simulink model "Octacopter_Model_24b"  (R2025b)
settings: Solver=VariableStepAuto  StartTime=0.0  StopTime=10  RelTol=1e-3
values from neighbouring files (symbols this model uses):
  Alt = 600    [Octa_Initialise.m]
  c = -500    [Octa_Initialise.m]
  Drag_on = 1    [Octa_Initialise.m]
  g = 9.81    [Octa_Initialise.m]
  I = [I_xx, I_xy, I_xz; I_xy, I_yy, I_yz; I_xz, I_yz, I_zz]    [Octa_Initialise.m]
  I_xx = 0.35    [Octa_Initialise.m]
  I_yy = 0.35    [Octa_Initialise.m]
  I_zz = 0.67    [Octa_Initialise.m]
  k = 6500    [Octa_Initialise.m]
  k_D = [0.05, 0.05, 0.15]    [Octa_Initialise.m]
  k_q = (Cp*Rho*(D)^5)/(8*(pi)^3)    (= 1.08765022525e-07)    [Octa_Initialise.m]
  l_arm1 = [l*cosd(0) l*sind(0) 0]    [Octa_Initialise.m]
  l_arm2 = [l*cosd(-45) l*sind(-45) 0]    [Octa_Initialise.m]
  l_arm3 = [l*cosd(-90) l*sind(-90) 0]    [Octa_Initialise.m]
  l_arm4 = [l*cosd(-135) l*sind(-135) 0]    [Octa_Initialise.m]
  l_arm5 = [l*cosd(-180) l*sind(-180) 0]    [Octa_Initialise.m]
  l_arm6 = [l*cosd(135) l*sind(135) 0]    [Octa_Initialise.m]
  l_arm7 = [l*cosd(90) l*sind(90) 0]    [Octa_Initialise.m]
  l_arm8 = [l*cosd(45) l*sind(45) 0]    [Octa_Initialise.m]
  m = 6.71    [Octa_Initialise.m]
  M1_set_phi = 0    [Octa_Initialise.m]
  M1_set_theta = 0    [Octa_Initialise.m]
  M2_set_phi = 0    [Octa_Initialise.m]
  M2_set_theta = 0    [Octa_Initialise.m]
  M3_set_phi = 0    [Octa_Initialise.m]
  M3_set_theta = 0    [Octa_Initialise.m]
  M4_set_phi = 0    [Octa_Initialise.m]
  M4_set_theta = 0    [Octa_Initialise.m]
  M5_set_phi = 0    [Octa_Initialise.m]
  M5_set_theta = 0    [Octa_Initialise.m]
  M6_set_phi = 0    [Octa_Initialise.m]
  M6_set_theta = 0    [Octa_Initialise.m]
  M7_set_phi = 0    [Octa_Initialise.m]
  M7_set_theta = 0    [Octa_Initialise.m]
  M8_set_phi = 0    [Octa_Initialise.m]
  M8_set_theta = 0    [Octa_Initialise.m]
  p_dot_dot_0 = 0    [Octa_Initialise.m]
  phi_dot_0 = phi_theta_psi_dot_0(1)    [Octa_Initialise.m]
  phi_lower = deg2rad(-180)    [Octa_Initialise.m]
  phi_upper = deg2rad(180)    [Octa_Initialise.m]
  psi_dot_0 = phi_theta_psi_dot_0(3)    [Octa_Initialise.m]
  q_dot_dot_0 = 0    [Octa_Initialise.m]
  r_dot_dot_0 = 0    [Octa_Initialise.m]
  rpm2rad_s = pi/30    (= 0.10471975512)    [Octa_Initialise.m]
  RPM_max = 17668    [Octa_Initialise.m]    (also in Thrust_Plots.m = 15000)
  RPM_min = 0    [Octa_Initialise.m]    (also in Thrust_Plots.m)
  Tau_ESC1 = 0.15    [Octa_Initialise.m]
  Tau_ESC2 = 0.15    [Octa_Initialise.m]
  Tau_ESC3 = 0.15    [Octa_Initialise.m]
  Tau_ESC4 = 0.15    [Octa_Initialise.m]
  Tau_ESC5 = 0.15    [Octa_Initialise.m]
  Tau_ESC6 = 0.15    [Octa_Initialise.m]
  Tau_ESC7 = 0.15    [Octa_Initialise.m]
  Tau_ESC8 = 0.15    [Octa_Initialise.m]
  theta_dot_0 = phi_theta_psi_dot_0(2)    [Octa_Initialise.m]
  theta_lower = deg2rad(-90)    [Octa_Initialise.m]
  theta_upper = deg2rad(90)    [Octa_Initialise.m]
  Thrust_max = 20    [Octa_Initialise.m]
  thrustData = load('Cine66 Thrust Params.mat')    [Thrust_Plots.m]
  u_0 = u_v_w_0(1)    [Octa_Initialise.m]
  u_dot_0 = 0    [Octa_Initialise.m]
  v_0 = u_v_w_0(2)    [Octa_Initialise.m]
  v_dot_0 = 0    [Octa_Initialise.m]
  w1_0 = 0    [Octa_Initialise.m]
  w2_0 = 0    [Octa_Initialise.m]
  w3_0 = 0    [Octa_Initialise.m]
  w4_0 = 0    [Octa_Initialise.m]
  w5_0 = 0    [Octa_Initialise.m]
  w6_0 = 0    [Octa_Initialise.m]
  w7_0 = 0    [Octa_Initialise.m]
  w8_0 = 0    [Octa_Initialise.m]
  w_0 = u_v_w_0(3)    [Octa_Initialise.m]
  w_d_1 = -1    [Octa_Initialise.m]
  w_d_2 = +1.    (= 1)    [Octa_Initialise.m]
  w_d_3 = -1    [Octa_Initialise.m]
  w_d_4 = +1    (= 1)    [Octa_Initialise.m]
  w_d_5 = -1    [Octa_Initialise.m]
  w_d_6 = +1    (= 1)    [Octa_Initialise.m]
  w_d_7 = -1    [Octa_Initialise.m]
  w_d_8 = +1    (= 1)    [Octa_Initialise.m]
  w_dot_0 = 0    [Octa_Initialise.m]
undefined symbols (not defined in the file or in its folder): DiscIntNeverNeededParam
libraries: matrix_library x10, simulink x3, px4uORBlib x1, aerolibutil x1, px4Peripheralslib x1
(part 1 of 2)
settings Model: PauseTimes=0.1  Creator=Admin  LastModifiedBy=Admin
settings DebuggingCC: AlgebraicLoopMsg=none

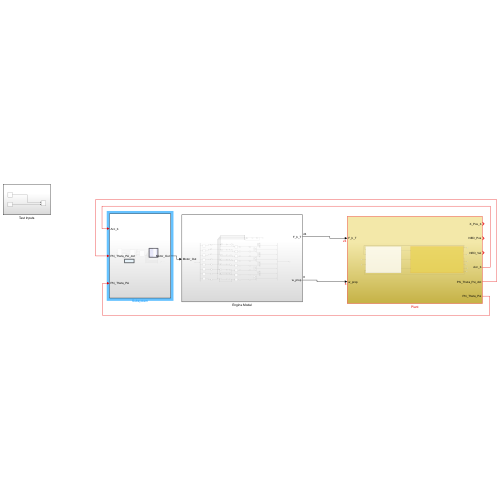
[thumbnail: Simulink's stored preview of the top-level diagram]
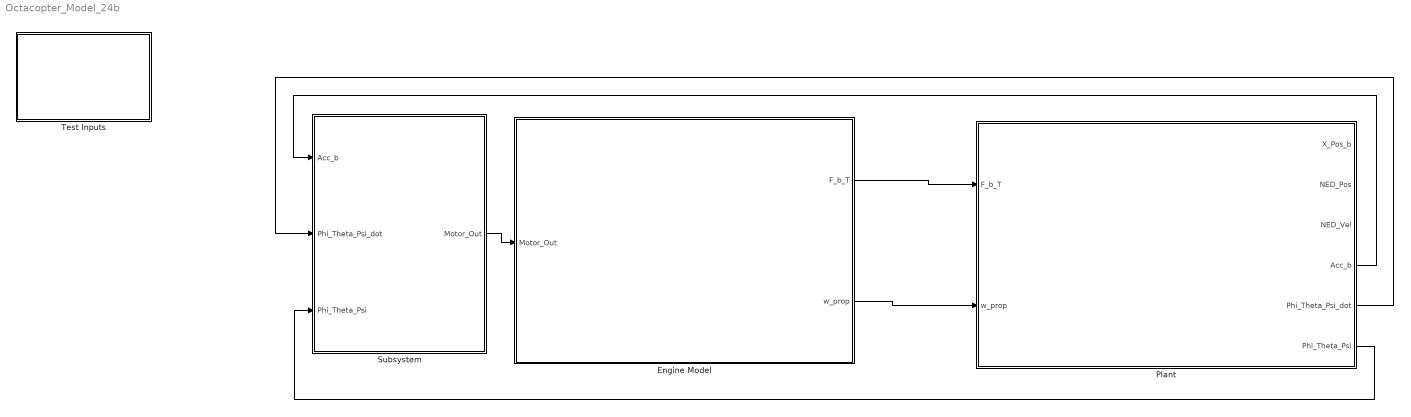
== system Octacopter_Model_24b ==
  Engine Model : Subsystem
  Plant : Subsystem
  Subsystem : Subsystem
  Test Inputs : Subsystem
  wires:
  Engine Model/1(F_b_T) -> Plant/1(F_b_T)
  Engine Model/2(w_prop) -> Plant/2(w_prop)
  Subsystem/1(Motor_Out) -> Engine Model/1(Motor_Out)
  Plant/4(Acc_b) -> Subsystem/1(Acc_b)
  Plant/5(Phi_Theta_Psi_dot) -> Subsystem/2(Phi_Theta_Psi_dot)
  Plant/6(Phi_Theta_Psi) -> Subsystem/3(Phi_Theta_Psi)

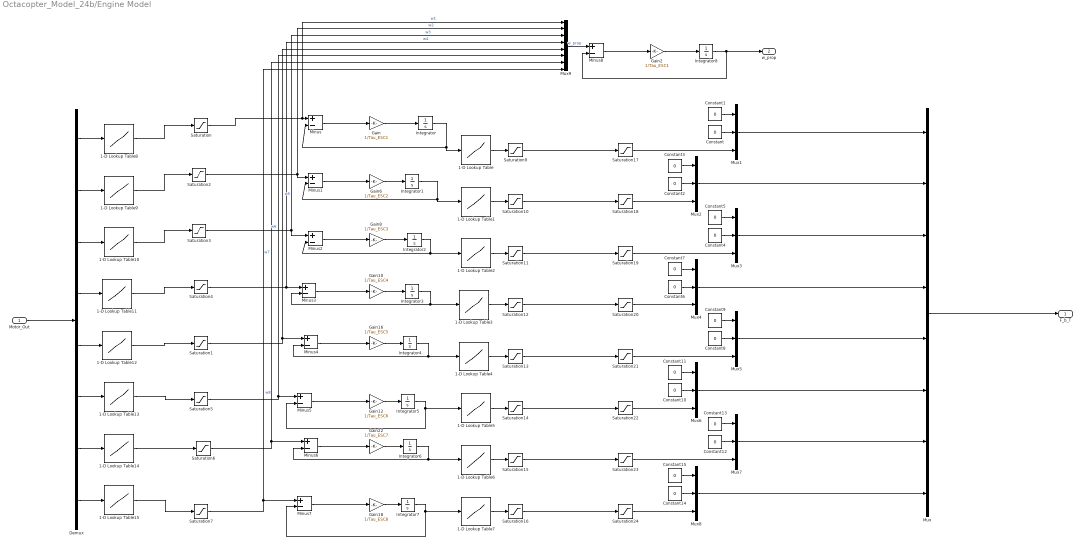
== system Octacopter_Model_24b/Engine Model ==
  Motor_Out : Inport
  1-D Lookup Table{,1..7} (8 alike) : Lookup_n-D  NumberOfTableDimensions=1  BreakpointsForDimension1=thrustData.RPM  Table=thrustData.Thrust_N_  InternalRulePriority=Speed  RndMeth=Simplest
  1-D Lookup Table{8..15} (8 alike) : Lookup_n-D  NumberOfTableDimensions=1  BreakpointsForDimension1=thrustData.Throttle  Table=thrustData.RPM  InternalRulePriority=Speed  RndMeth=Simplest
  Constant{,1..15} (16 alike) : Constant  Value=0
  Demux : Demux  Outputs=8
  Gain : Gain  Gain=1/Tau_ESC1
  Gain10 : Gain  Gain=1/Tau_ESC4
  Gain12 : Gain  Gain=1/Tau_ESC6
  Gain16 : Gain  Gain=1/Tau_ESC5
  Gain18 : Gain  Gain=1/Tau_ESC8
  Gain2 : Gain  Gain=1/Tau_ESC1
  Gain22 : Gain  Gain=1/Tau_ESC7
  Gain6 : Gain  Gain=1/Tau_ESC2
  Gain8 : Gain  Gain=1/Tau_ESC3
  Integrator : Integrator  InitialCondition=w1_0
  Integrator1 : Integrator  InitialCondition=w2_0
  Integrator2 : Integrator  InitialCondition=w3_0
  Integrator3 : Integrator  InitialCondition=w4_0
  Integrator4 : Integrator  InitialCondition=w5_0
  Integrator5 : Integrator  InitialCondition=w6_0
  Integrator6 : Integrator  InitialCondition=w7_0
  Integrator7 : Integrator  InitialCondition=w8_0
  Integrator8 : Integrator  InitialCondition=w1_0
  Minus{,1..8} (9 alike) : Sum  Inputs=+-
  Mux : Mux  Inputs=8
  Mux{1..8} (8 alike) : Mux  Inputs=3
  Mux9 : Mux  Inputs=8
  Saturation{,1..7} (8 alike) : Saturate  UpperLimit=RPM_max  LowerLimit=RPM_min
  Saturation{9..24} (16 alike) : Saturate  UpperLimit=Thrust_max  LowerLimit=0
  F_b_T : Outport
  w_prop : Outport  Port=2
  wires:
  Minus/1 -> Gain/1
  Gain/1 -> Integrator/1
  Mux/1 -> F_b_T/1
  Gain6/1 -> Integrator1/1
  Minus1/1 -> Gain6/1
  Gain8/1 -> Integrator2/1
  Minus2/1 -> Gain8/1
  Minus3/1 -> Gain10/1
  Gain10/1 -> Integrator3/1
  1-D Lookup Table/1 -> Saturation9/1
  1-D Lookup Table1/1 -> Saturation10/1
  1-D Lookup Table2/1 -> Saturation11/1
  1-D Lookup Table3/1 -> Saturation12/1
  Saturation9/1 -> Saturation17/1
  Integrator/1 -> Minus/2, 1-D Lookup Table/1
  Integrator1/1 -> 1-D Lookup Table1/1, Minus1/2
  Integrator2/1 -> 1-D Lookup Table2/1, Minus2/2
  Integrator3/1 -> 1-D Lookup Table3/1, Minus3/2
  Integrator5/1 -> 1-D Lookup Table5/1, Minus5/2
  Integrator4/1 -> 1-D Lookup Table4/1, Minus4/2
  1-D Lookup Table5/1 -> Saturation14/1
  1-D Lookup Table4/1 -> Saturation13/1
  Gain12/1 -> Integrator5/1
  Minus5/1 -> Gain12/1
  Minus4/1 -> Gain16/1
  Gain16/1 -> Integrator4/1
  Gain22/1 -> Integrator6/1
  Minus6/1 -> Gain22/1
  Minus7/1 -> Gain18/1
  Gain18/1 -> Integrator7/1
  1-D Lookup Table6/1 -> Saturation15/1
  1-D Lookup Table7/1 -> Saturation16/1
  Integrator6/1 -> 1-D Lookup Table6/1, Minus6/2
  Integrator7/1 -> 1-D Lookup Table7/1, Minus7/2
  Constant1/1 -> Mux1/1
  Constant/1 -> Mux1/2
  Constant2/1 -> Mux2/2
  Constant3/1 -> Mux2/1
  Saturation10/1 -> Saturation18/1
  Constant4/1 -> Mux3/2
  Saturation11/1 -> Saturation19/1
  Constant5/1 -> Mux3/1
  Constant6/1 -> Mux4/2
  Saturation12/1 -> Saturation20/1
  Constant7/1 -> Mux4/1
  Constant8/1 -> Mux5/2
  Saturation13/1 -> Saturation21/1
  Constant9/1 -> Mux5/1
  Constant10/1 -> Mux6/2
  Saturation14/1 -> Saturation22/1
  Constant11/1 -> Mux6/1
  Constant12/1 -> Mux7/2
  Saturation15/1 -> Saturation23/1
  Constant13/1 -> Mux7/1
  Constant14/1 -> Mux8/2
  Saturation16/1 -> Saturation24/1
  Constant15/1 -> Mux8/1
  Mux1/1 -> Mux/1
  Mux2/1 -> Mux/2
  Mux3/1 -> Mux/3
  Mux4/1 -> Mux/4
  Mux5/1 -> Mux/5
  Mux6/1 -> Mux/6
  Mux7/1 -> Mux/7
  Mux8/1 -> Mux/8
  Saturation17/1 -> Mux1/3
  Saturation18/1 -> Mux2/3
  Saturation19/1 -> Mux3/3
  Saturation20/1 -> Mux4/3
  Saturation21/1 -> Mux5/3
  Saturation22/1 -> Mux6/3
  Saturation23/1 -> Mux7/3
  Saturation24/1 -> Mux8/3
  Saturation/1 -> Mux9/1, Minus/1  "w1"
  Saturation2/1 -> Mux9/2, Minus1/1  "w2"
  Saturation3/1 -> Mux9/3, Minus2/1  "w3"
  Saturation4/1 -> Mux9/4, Minus3/1  "w4"
  Saturation7/1 -> Mux9/8, Minus7/1  "w8"
  Saturation6/1 -> Mux9/7, Minus6/1  "w7"
  Saturation5/1 -> Mux9/6, Minus5/1  "w6"
  Saturation1/1 -> Mux9/5, Minus4/1  "w5"
  Mux9/1 -> Minus8/1  "w_prop"
  Integrator8/1 -> Minus8/2, w_prop/1
  Minus8/1 -> Gain2/1
  Gain2/1 -> Integrator8/1
  1-D Lookup Table8/1 -> Saturation/1
  1-D Lookup Table9/1 -> Saturation2/1
  1-D Lookup Table10/1 -> Saturation3/1
  1-D Lookup Table11/1 -> Saturation4/1
  1-D Lookup Table12/1 -> Saturation1/1
  1-D Lookup Table13/1 -> Saturation5/1
  1-D Lookup Table14/1 -> Saturation6/1
  1-D Lookup Table15/1 -> Saturation7/1
  Demux/1 -> 1-D Lookup Table8/1
  Demux/2 -> 1-D Lookup Table9/1
  Demux/3 -> 1-D Lookup Table10/1
  Demux/4 -> 1-D Lookup Table11/1
  Demux/5 -> 1-D Lookup Table12/1
  Demux/6 -> 1-D Lookup Table13/1
  Demux/7 -> 1-D Lookup Table14/1
  Demux/8 -> 1-D Lookup Table15/1
  Motor_Out/1 -> Demux/1

== system Octacopter_Model_24b/Plant ==
  F_b_T : Inport
  w_prop : Inport  Port=2
  EOM : Subsystem
  Force & Moments : Subsystem
  X_Pos_b : Outport
  NED_Pos : Outport  Port=2
  NED_Vel : Outport  Port=3
  Acc_b : Outport  Port=4
  Phi_Theta_Psi_dot : Outport  Port=5
  Phi_Theta_Psi : Outport  Port=6
  wires:
  Force & Moments/1(M_b_tot) -> EOM/1(M_b_Tot)  "M_b_Tot"
  EOM/1(Phi_Theta_Psi) -> Phi_Theta_Psi/1, Force & Moments/1(w (PhiThetaPsi))
  EOM/2(V_i (uvw)) -> Force & Moments/2(V_i (uvw))
  Force & Moments/2(F_ext_b_Tot) -> EOM/2(F_ext_b_Tot)
  w_prop/1 -> Force & Moments/4(w_prop)
  Force & Moments/3(T_F_b) -> EOM/3(T_F_b)
  EOM/4(On_Grnd) -> Force & Moments/5(Ldg_Param)
  F_b_T/1 -> Force & Moments/3(F_b_T)
  EOM/3(X_Pos_b) -> X_Pos_b/1
  EOM/5(NED_Pos) -> NED_Pos/1
  EOM/6(NED_Vel) -> NED_Vel/1
  EOM/7(Acc_b) -> Acc_b/1
  EOM/8(Phi_Theta_Psi_dot) -> Phi_Theta_Psi_dot/1

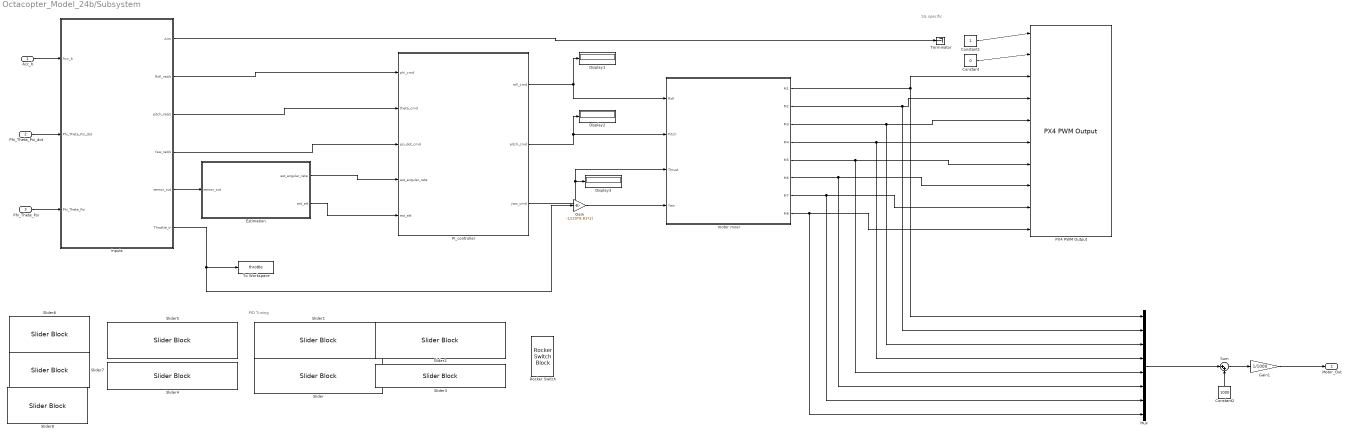
== system Octacopter_Model_24b/Subsystem ==
  note: SIL specific
  note: PID Tuning
  Acc_b : Inport
  Phi_Theta_Psi_dot : Inport  Port=2
  Phi_Theta_Psi : Inport  Port=3
  Constant : Constant  Value=0  OutDataTypeStr=boolean
  Constant1 : Constant  OutDataTypeStr=boolean
  Constant2 : Constant  Value=1000
  Display1 : Display
  Display2 : Display
  Display3 : Display
  Estimation : Subsystem
  Gain : Gain  Gain=-1/(20*9.81*2)
  Gain1 : Gain  Gain=1/1000
  Inputs : Subsystem
  Mux : Mux  Inputs=8
  "PI_controller " : Subsystem
  PX4 PWM Output : px4Peripheralslib/PX4 PWM Output  pwmDevice=Main  pwmChannel1_=on  pwmChannel2_=on  pwmChannel3_=on  pwmChannel4_=on  pwmChannel5_=on  pwmChannel6_=on  pwmChannel7_=on  pwmChannel8_=on
  Rocker Switch : RockerSwitchBlock
  Slider : SliderBlock  ScaleMax=0.1
  Slider1 : SliderBlock  ScaleMax=0.5
  Slider2 : SliderBlock  ScaleMax=0.5
  Slider3 : SliderBlock  ScaleMax=0.1
  Slider4 : SliderBlock  ScaleMax=1
  Slider5 : SliderBlock  ScaleMax=1
  Slider6 : SliderBlock  ScaleMax=5
  Slider7 : SliderBlock  ScaleMax=5
  Slider8 : SliderBlock  ScaleMax=5
  Sum : Sum  Inputs=|++
  Terminator : Terminator
  To Workspace : ToWorkspace  VariableName=throttle  SaveFormat=Structure With Time  SampleTime=-1
  motor mxer : MATLAB Function  TreatAsAtomicUnit=on
  Motor_Out : Outport
  wires:
  Inputs/1(Arm) -> Terminator/1
  "PI_controller "/3(yaw_cmd) -> motor mxer/3(Thrust), Display3/1
  motor mxer/5(M5) -> Mux/5, PX4 PWM Output/7
  motor mxer/1(M1) -> Mux/1, PX4 PWM Output/3
  Inputs/6(Throttle_in) -> Gain/1, To Workspace/1
  Inputs/4(Yaw_rad/s) -> "PI_controller "/3(psi_dot_cmd)
  Inputs/3(pitch_rad/s) -> "PI_controller "/2(theta_cmd)
  Inputs/5(sensor_out) -> Estimation/1(sensor_out)
  Gain/1 -> motor mxer/4(Yaw)
  "PI_controller "/2(pitch_cmd) -> motor mxer/2(Pitch), Display2/1
  motor mxer/2(M2) -> Mux/2, PX4 PWM Output/4
  motor mxer/3(M3) -> Mux/3, PX4 PWM Output/5
  Estimation/1(est_angular_rate) -> "PI_controller "/4(est_angular_rate)
  "PI_controller "/1(roll_cmd) -> Display1/1, motor mxer/1(Roll)
  motor mxer/4(M4) -> Mux/4, PX4 PWM Output/6
  Constant/1 -> PX4 PWM Output/2
  Estimation/2(est_att) -> "PI_controller "/5(est_att)
  motor mxer/6(M6) -> Mux/6, PX4 PWM Output/8
  motor mxer/8(M8) -> Mux/8, PX4 PWM Output/10
  Inputs/2(Roll_rad/s) -> "PI_controller "/1(phi_cmd)
  Constant1/1 -> PX4 PWM Output/1
  motor mxer/7(M7) -> Mux/7, PX4 PWM Output/9
  Mux/1 -> Sum/1
  Constant2/1 -> Sum/2
  Sum/1 -> Gain1/1
  Gain1/1 -> Motor_Out/1
  Acc_b/1 -> Inputs/1(Acc_b)
  Phi_Theta_Psi_dot/1 -> Inputs/2(Phi_Theta_Psi_dot)
  Phi_Theta_Psi/1 -> Inputs/3(Phi_Theta_Psi)

== system Octacopter_Model_24b/Test Inputs ==
  Pulse Generator : DiscretePulseGenerator  PulseType=Time based  Amplitude=0.7  Period=50  PulseWidth=50
  Scope : Scope  NumInputPorts=2
      settings: ActiveDisplayYMinimum=-0.087499999999999981  ActiveDisplayYMaximum=0.7875  DataLoggingVariableName=ScopeData7
  Step : Step  Time=2  After=0.69  SampleTime=30
  wires:
  Pulse Generator/1 -> Scope/1
  Step/1 -> Scope/2

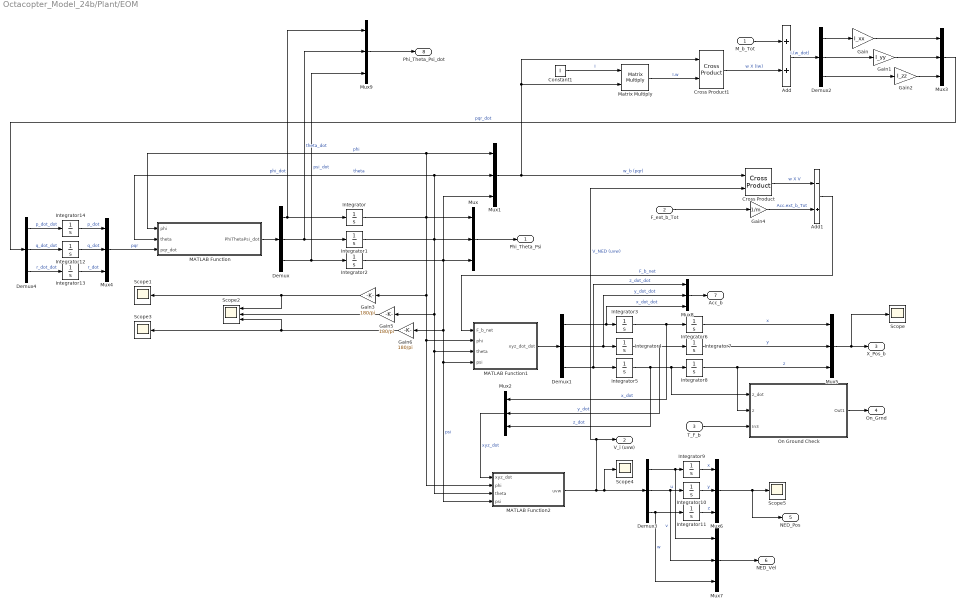
== system Octacopter_Model_24b/Plant/EOM ==
  M_b_Tot : Inport
  F_ext_b_Tot : Inport  Port=2
  T_F_b : Inport  Port=3
  Add : Sum
  Add1 : Sum  Inputs=-+
  Constant1 : Constant  Value=I
  Cross Product : matrix_library/Cross Product
  Cross Product1 : matrix_library/Cross Product
  Demux{,1..4} (5 alike) : Demux  Outputs=3
  Gain : Gain  Gain=I_xx
  Gain1 : Gain  Gain=I_yy
  Gain2 : Gain  Gain=I_zz
  Gain3 : Gain  Gain=180/pi
  Gain4 : Gain  Gain=1/m
  Gain5 : Gain  Gain=180/pi
  Gain6 : Gain  Gain=180/pi
  Integrator : Integrator  InitialCondition=phi_dot_0  LimitOutput=on  UpperSaturationLimit=phi_upper  LowerSaturationLimit=phi_lower  WrappedStateUpperValue=phi_upper  WrappedStateLowerValue=phi_lower
  Integrator1 : Integrator  InitialCondition=theta_dot_0  LimitOutput=on  UpperSaturationLimit=theta_upper  LowerSaturationLimit=theta_lower  WrappedStateUpperValue=theta_upper  WrappedStateLowerValue=theta_lower
  Integrator10 : Integrator  InitialCondition=v_0
  Integrator11 : Integrator  InitialCondition=w_0  LowerSaturationLimit=Alt-1
  Integrator12 : Integrator  InitialCondition=q_dot_dot_0
  Integrator13 : Integrator  InitialCondition=r_dot_dot_0
  Integrator14 : Integrator  InitialCondition=p_dot_dot_0
  Integrator2 : Integrator  InitialCondition=psi_dot_0  WrapState=on  WrappedStateUpperValue=psi_upper  WrappedStateLowerValue=psi_lower
  Integrator3 : Integrator  InitialCondition=u_dot_0
  Integrator4 : Integrator  InitialCondition=v_dot_0
  Integrator5 : Integrator  InitialCondition=-w_dot_0
  Integrator6 : Integrator  InitialCondition=u_0
  Integrator7 : Integrator  InitialCondition=v_0
  Integrator8 : Integrator  InitialCondition=w_0  LowerSaturationLimit=Alt-1
  Integrator9 : Integrator  InitialCondition=u_0
  MATLAB Function : MATLAB Function  TreatAsAtomicUnit=on
  MATLAB Function1 : MATLAB Function  TreatAsAtomicUnit=on
  MATLAB Function2 : MATLAB Function  TreatAsAtomicUnit=on
  Matrix Multiply : Product  Multiplication=Matrix(*)
  Mux{,1..9} (10 alike) : Mux  Inputs=3
  On Ground Check : Subsystem
  Scope{,1,3..5} (5 alike) : Scope
      Scope settings: ActiveDisplayYMinimum=-142.301718259967  ActiveDisplayYMaximum=1280.7154643397032
      Scope1 settings: ActiveDisplayYMinimum=-0.95325786516340649  ActiveDisplayYMaximum=7.8270007011494336
      Scope3 settings: ActiveDisplayYMinimum=-1  ActiveDisplayYMaximum=1  DataLoggingVariableName=ScopeData3
      Scope4 settings: ActiveDisplayYMinimum=-102.25832715751218  ActiveDisplayYMaximum=917.59584332329212  DataLoggingVariableName=ScopeData4
      Scope5 settings: ActiveDisplayYMinimum=-102.25832715751218  ActiveDisplayYMaximum=917.59584332329212  DataLoggingVariableName=ScopeData5
  Scope2 : Scope  NumInputPorts=3
      settings: ActiveDisplayYMinimum=-1.7055556366273353E-12  ActiveDisplayYMaximum=2.4470577937507177E-12  DataLoggingVariableName=ScopeData2
  Phi_Theta_Psi : Outport
  V_i (uvw) : Outport  Port=2
  X_Pos_b : Outport  Port=3
  On_Grnd : Outport  Port=4
  NED_Pos : Outport  Port=5
  NED_Vel : Outport  Port=6
  Acc_b : Outport  Port=7
  Phi_Theta_Psi_dot : Outport  Port=8
  wires:
  Integrator2/1 -> Mux/3, Mux1/3, Gain6/1, MATLAB Function1/4(psi), MATLAB Function2/4(psi)  "psi"
  Gain4/1 -> Add1/2  "Acc.ext_b_Tot"
  Mux1/1 -> Cross Product/1, Cross Product1/1, Matrix Multiply/2  "w_b (pqr)"
  Mux4/1 -> MATLAB Function/3(pqr_dot)  "pqr"
  Demux4/2 -> Integrator12/1  "q_dot_dot"
  Integrator/1 -> Mux/1, Mux1/1, MATLAB Function/1(phi), MATLAB Function2/2(phi), MATLAB Function1/2(phi), Gain3/1  "phi"
  Add/1 -> Demux2/1  "I.(w_dot)"
  Gain2/1 -> Mux3/3
  Demux/3 -> Integrator2/1, Mux9/3  "psi_dot"
  Gain/1 -> Mux3/1
  Integrator1/1 -> Mux/2, MATLAB Function1/3(theta), MATLAB Function2/3(theta), Gain5/1, Mux1/2, MATLAB Function/2(theta)  "theta"
  Demux/1 -> Mux9/1, Integrator/1  "phi_dot"
  MATLAB Function1/1(xyz_dot_dot) -> Demux1/1
  Integrator13/1 -> Mux4/3  "r_dot"
  Add1/1 -> MATLAB Function1/1(F_b_net)  "F_b_net"
  M_b_Tot/1 -> Add/1
  MATLAB Function2/1(uvw) -> V_i (uvw)/1, Cross Product/2, Scope4/1, Demux3/1  "V_NED (uvw)"
  Demux2/1 -> Gain/1
  Demux2/2 -> Gain1/1
  Integrator12/1 -> Mux4/2  "q_dot"
  Demux/2 -> Mux9/2, Integrator1/1  "theta_dot"
  Integrator14/1 -> Mux4/1  "p_dot"
  Matrix Multiply/1 -> Cross Product1/2  "I.w"
  Mux3/1 -> Demux4/1  "pqr_dot"
  Demux4/3 -> Integrator13/1  "r_dot_dot"
  MATLAB Function/1(PhiThetaPsi_dot) -> Demux/1
  Mux2/1 -> MATLAB Function2/1(xyz_dot)  "xyz_dot"
  Demux2/3 -> Gain2/1
  Gain1/1 -> Mux3/2
  Constant1/1 -> Matrix Multiply/1  "I"
  Cross Product/1 -> Add1/1  "w X V"
  Demux1/3 -> Mux8/1, Integrator5/1  "z_dot_dot"
  Cross Product1/1 -> Add/2  "w X (Iw)"
  Demux4/1 -> Integrator14/1  "p_dot_dot"
  F_ext_b_Tot/1 -> Gain4/1
  Mux/1 -> Phi_Theta_Psi/1
  Mux5/1 -> X_Pos_b/1, Scope/1
  Demux1/1 -> Mux8/3, Integrator3/1  "x_dot_dot"
  Integrator5/1 -> Mux2/3, On Ground Check/1(z_dot), Integrator8/1  "z_dot"
  Integrator3/1 -> Integrator6/1, Mux2/1  "x_dot"
  Integrator4/1 -> Mux2/2, Integrator7/1  "y_dot"
  Integrator6/1 -> Mux5/1  "x"
  Integrator7/1 -> Mux5/2  "y"
  Demux1/2 -> Mux8/2, Integrator4/1  "y_dot_dot"
  Gain3/1 -> Scope2/1, Scope1/1
  Gain5/1 -> Scope2/2
  Gain6/1 -> Scope2/3, Scope3/1
  Integrator8/1 -> Mux5/3, On Ground Check/2(z)  "z"
  T_F_b/1 -> On Ground Check/3(In3)
  On Ground Check/1(Out1) -> On_Grnd/1
  Demux3/2 -> Mux7/2, Integrator10/1  "v"
  Demux3/1 -> Mux7/1, Integrator9/1  "u"
  Demux3/3 -> Mux7/3, Integrator11/1  "w"
  Integrator9/1 -> Mux6/1  "x"
  Integrator10/1 -> Mux6/2  "y"
  Integrator11/1 -> Mux6/3  "z"
  Mux6/1 -> NED_Pos/1, Scope5/1
  Mux7/1 -> NED_Vel/1
  Mux8/1 -> Acc_b/1
  Mux9/1 -> Phi_Theta_Psi_dot/1

== system Octacopter_Model_24b/Plant/Force & Moments ==
  w (PhiThetaPsi) : Inport
  V_i (uvw) : Inport  Port=2
  F_b_T : Inport  Port=3
  w_prop : Inport  Port=4
  Ldg_Param : Inport  Port=5
  Other Forces : Subsystem
  Thrust Forces and Moments : Subsystem
  M_b_tot : Outport
  F_ext_b_Tot : Outport  Port=2
  T_F_b : Outport  Port=3
  wires:
  w (PhiThetaPsi)/1 -> Other Forces/2(w (PhiThetaPsi))
  V_i (uvw)/1 -> Other Forces/3(V_i)
  Ldg_Param/1 -> Other Forces/4(In4)
  Other Forces/2(F_ext_b_Tot) -> F_ext_b_Tot/1
  w_prop/1 -> Thrust Forces and Moments/1(w_prop)
  F_b_T/1 -> Thrust Forces and Moments/2(F_b_T)
  Other Forces/1(F_b_D) -> Thrust Forces and Moments/3(In3)
  Thrust Forces and Moments/1(M_b_tot) -> M_b_tot/1
  Thrust Forces and Moments/2(T_F_b) -> T_F_b/1, Other Forces/1(T_F_b)

== system Octacopter_Model_24b/Subsystem/Estimation ==
  sensor_out : Inport
  Bus Creator : BusCreator  Inputs=3
  Bus Selector : BusSelector  OutputSignals=w_x_meas,w_y_meas,w_z_meas
  Bus Selector1 : BusSelector  OutputSignals=roll_meas,pitch_meas,yaw_meas
  Saturation : Saturate  UpperLimit=0.70  LowerLimit=-0.70
  Saturation1 : Saturate  UpperLimit=0.70  LowerLimit=-0.70
  Saturation2 : Saturate  UpperLimit=3.14  LowerLimit=-3.14
  Subsystem3 : Subsystem
  est_angular_rate : Outport
  est_att : Outport  Port=2
  wires:
  Subsystem3/1(est_angular_rate) -> est_angular_rate/1
  sensor_out/1 -> Bus Selector1/1, Bus Selector/1
  Bus Selector/1 -> Subsystem3/1(In1)  "<w_x_meas>"
  Bus Selector/2 -> Subsystem3/2(In2)  "<w_y_meas>"
  Bus Selector/3 -> Subsystem3/3(In3)  "<w_z_meas>"
  Bus Selector1/1 -> Saturation/1  "<roll_meas>"
  Bus Selector1/2 -> Saturation1/1  "<pitch_meas>"
  Bus Selector1/3 -> Saturation2/1  "<yaw_meas>"
  Saturation1/1 -> Bus Creator/2  "pitch"
  Saturation/1 -> Bus Creator/1  "roll"
  Saturation2/1 -> Bus Creator/3  "yaw"
  Bus Creator/1 -> est_att/1

== system Octacopter_Model_24b/Subsystem/Inputs ==
  Acc_b : Inport
  Phi_Theta_Psi_dot : Inport  Port=2
  Phi_Theta_Psi : Inport  Port=3
  RC_input : Subsystem
  Sensors_meas : Subsystem
  Stick_mapping : Subsystem
  Arm : Outport
  Roll_rad/s : Outport  Port=2
  pitch_rad/s : Outport  Port=3
  Yaw_rad/s : Outport  Port=4
  sensor_out : Outport  Port=5
  Throttle_in : Outport  Port=6
  wires:
  Sensors_meas/1(sensor_out) -> sensor_out/1
  RC_input/1(Arm) -> Arm/1
  RC_input/2(Roll_in) -> Stick_mapping/1(Roll_in)
  RC_input/3(Pitch_in) -> Stick_mapping/2(Pitch_in)
  RC_input/4(Throttle_in) -> Stick_mapping/3(Throttle_in)
  RC_input/5(Yaw_in) -> Stick_mapping/4(yaw_in)
  Stick_mapping/1(Roll_rad) -> Roll_rad/s/1
  Stick_mapping/2(Pitch_rad) -> pitch_rad/s/1
  Stick_mapping/3(Throttle) -> Throttle_in/1
  Stick_mapping/4(yaw_rad/s) -> Yaw_rad/s/1
  Phi_Theta_Psi_dot/1 -> Sensors_meas/2(Phi_Theta_Psi_dot)
  Phi_Theta_Psi/1 -> Sensors_meas/3(Phi_Theta_Psi)
  Acc_b/1 -> Sensors_meas/1(Acc_b)

== system Octacopter_Model_24b/Subsystem/PI_controller  ==
  phi_cmd : Inport
  theta_cmd : Inport  Port=2
  psi_dot_cmd : Inport  Port=3
  est_angular_rate : Inport  Port=4
  est_att : Inport  Port=5
  Subsystem : Subsystem
  rotational : Subsystem
  roll_cmd : Outport
  pitch_cmd : Outport  Port=2
  yaw_cmd : Outport  Port=3
  wires:
  phi_cmd/1 -> Subsystem/1(phi_cmd)
  theta_cmd/1 -> Subsystem/2(theta_cmd)
  psi_dot_cmd/1 -> Subsystem/3(psi_cmd)
  est_att/1 -> Subsystem/4(est_att)
  est_angular_rate/1 -> rotational/4(est_angular_rate)
  Subsystem/1(p_cmd) -> rotational/1(p_cmd)
  Subsystem/2(q_cmd) -> rotational/2(q_cmd)
  Subsystem/3(r_dot_cmd) -> rotational/3(r_dot_cmd)
  rotational/1(P_dot) -> roll_cmd/1
  rotational/2(q_dot) -> pitch_cmd/1
  rotational/3(r_dot) -> yaw_cmd/1

== system Octacopter_Model_24b/Plant/EOM/On Ground Check ==
  z_dot : Inport
  z : Inport  Port=2
  In3 : Inport  Port=3
  AND : Logic  IconShape=distinctive  AllPortsSameDT=off  OutDataTypeStr=boolean
  Compare To Constant : simulink/Logic and Bit Operations/Compare To Constant  relop=<  const=Alt  OutDataTypeStr=boolean
  Compare To Constant1 : simulink/Logic and Bit Operations/Compare To Constant  relop=<=  const=m*g  OutDataTypeStr=boolean
  Data Type Conversion : DataTypeConversion  OutDataTypeStr=double  SaturateOnIntegerOverflow=off  RndMeth=Floor
  Demux3 : Demux  Outputs=3
  Mux6 : Mux  Inputs=3
  Terminator : Terminator
  Terminator1 : Terminator
  Out1 : Outport
  wires:
  z/1 -> Compare To Constant/1, Mux6/1
  Compare To Constant/1 -> AND/1
  Demux3/1 -> Terminator/1
  AND/1 -> Data Type Conversion/1
  Mux6/1 -> Out1/1
  Compare To Constant1/1 -> AND/2
  Demux3/3 -> Compare To Constant1/1
  Demux3/2 -> Terminator1/1
  Data Type Conversion/1 -> Mux6/3
  z_dot/1 -> Mux6/2
  In3/1 -> Demux3/1

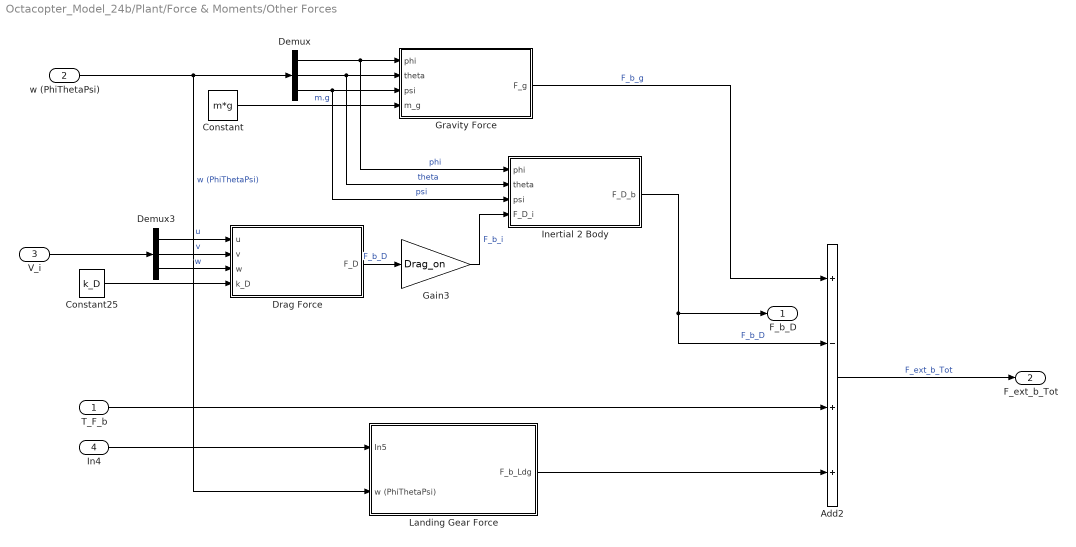
== system Octacopter_Model_24b/Plant/Force & Moments/Other Forces ==
  T_F_b : Inport
  w (PhiThetaPsi) : Inport  Port=2
  V_i : Inport  Port=3
  In4 : Inport  Port=4
  Add2 : Sum  Inputs=+-++
  Constant : Constant  Value=m*g
  Constant25 : Constant  Value=k_D
  Demux : Demux  Outputs=3
  Demux3 : Demux  Outputs=3
  Drag Force : MATLAB Function  TreatAsAtomicUnit=on
  Gain3 : Gain  Gain=Drag_on
  Gravity Force : MATLAB Function  TreatAsAtomicUnit=on
  Inertial 2 Body : MATLAB Function  TreatAsAtomicUnit=on
  Landing Gear Force : Subsystem
  F_b_D : Outport
  F_ext_b_Tot : Outport  Port=2
  wires:
  Constant/1 -> Gravity Force/4(m_g)  "m.g"
  w (PhiThetaPsi)/1 -> Landing Gear Force/2(w (PhiThetaPsi)), Demux/1  "w (PhiThetaPsi)"
  Constant25/1 -> Drag Force/4(k_D)
  Demux/1 -> Gravity Force/1(phi), Inertial 2 Body/1(phi)  "phi"
  Demux3/3 -> Drag Force/3(w)  "w"
  Gain3/1 -> Inertial 2 Body/4(F_D_i)  "F_b_i"
  Demux/3 -> Inertial 2 Body/3(psi), Gravity Force/3(psi)  "psi"
  Landing Gear Force/1(F_b_Ldg) -> Add2/4
  Drag Force/1(F_D) -> Gain3/1  "F_b_D"
  Demux/2 -> Gravity Force/2(theta), Inertial 2 Body/2(theta)  "theta"
  Demux3/2 -> Drag Force/2(v)  "v"
  Gravity Force/1(F_g) -> Add2/1  "F_b_g"
  Demux3/1 -> Drag Force/1(u)  "u"
  In4/1 -> Landing Gear Force/1(In5)
  T_F_b/1 -> Add2/3
  Add2/1 -> F_ext_b_Tot/1  "F_ext_b_Tot"
  V_i/1 -> Demux3/1
  Inertial 2 Body/1(F_D_b) -> Add2/2, F_b_D/1  "F_b_D"

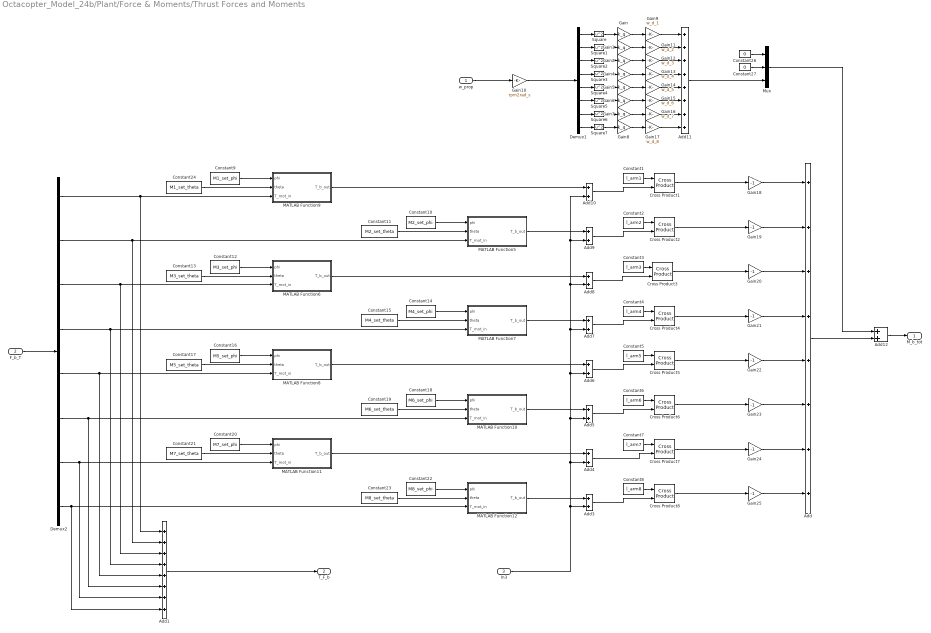
== system Octacopter_Model_24b/Plant/Force & Moments/Thrust Forces and Moments ==
  w_prop : Inport
  F_b_T : Inport  Port=2
  In3 : Inport  Port=3
  Add : Sum  Inputs=++++++++
  Add1 : Sum  Inputs=++++++++
  Add{3..10,12} (9 alike) : Sum
  Add11 : Sum  Inputs=++++++++
  Constant1 : Constant  Value=l_arm1
  Constant10 : Constant  Value=M2_set_phi
  Constant11 : Constant  Value=M2_set_theta
  Constant12 : Constant  Value=M3_set_phi
  Constant13 : Constant  Value=M3_set_theta
  Constant14 : Constant  Value=M4_set_phi
  Constant15 : Constant  Value=M4_set_theta
  Constant16 : Constant  Value=M5_set_phi
  Constant17 : Constant  Value=M5_set_theta
  Constant18 : Constant  Value=M6_set_phi
  Constant19 : Constant  Value=M6_set_theta  VectorParams1D=off
  Constant2 : Constant  Value=l_arm2
  Constant20 : Constant  Value=M7_set_phi
  Constant21 : Constant  Value=M7_set_theta
  Constant22 : Constant  Value=M8_set_phi
  Constant23 : Constant  Value=M8_set_theta
  Constant24 : Constant  Value=M1_set_theta
  Constant26 : Constant  Value=0
  Constant27 : Constant  Value=0
  Constant3 : Constant  Value=l_arm3
  Constant4 : Constant  Value=l_arm4
  Constant5 : Constant  Value=l_arm5
  Constant6 : Constant  Value=l_arm6
  Constant7 : Constant  Value=l_arm7
  Constant8 : Constant  Value=l_arm8
  Constant9 : Constant  Value=M1_set_phi
  Cross Product{1..8} (8 alike) : matrix_library/Cross Product
  Demux1 : Demux  Outputs=8
  Demux2 : Demux  Outputs=8
  Gain{,1..2,4..8} (8 alike) : Gain  Gain=k_q
  Gain10 : Gain  Gain=rpm2rad_s
  Gain11 : Gain  Gain=w_d_2
  Gain12 : Gain  Gain=w_d_3
  Gain13 : Gain  Gain=w_d_4
  Gain14 : Gain  Gain=w_d_5
  Gain15 : Gain  Gain=w_d_6
  Gain16 : Gain  Gain=w_d_7
  Gain17 : Gain  Gain=w_d_8
  Gain{18..25} (8 alike) : Gain  Gain=-1
  Gain9 : Gain  Gain=w_d_1
  MATLAB Function10 : MATLAB Function  TreatAsAtomicUnit=on
  MATLAB Function11 : MATLAB Function  TreatAsAtomicUnit=on
  MATLAB Function12 : MATLAB Function  TreatAsAtomicUnit=on
  MATLAB Function5 : MATLAB Function  TreatAsAtomicUnit=on
  MATLAB Function6 : MATLAB Function  TreatAsAtomicUnit=on
  MATLAB Function7 : MATLAB Function  TreatAsAtomicUnit=on
  MATLAB Function8 : MATLAB Function  TreatAsAtomicUnit=on
  MATLAB Function9 : MATLAB Function  TreatAsAtomicUnit=on
  Mux : Mux  Inputs=3
  Square{,1..7} (8 alike) : Math  Operator=square
  M_b_tot : Outport
  T_F_b : Outport  Port=2
  wires:
  In3/1 -> Add3/2, Add4/2, Add5/2, Add6/2, Add7/2, Add8/2, Add9/2, Add10/2
  Demux2/4 -> Add1/4, MATLAB Function7/3(T_mot_in)
  Demux2/5 -> Add1/5, MATLAB Function8/3(T_mot_in)
  Add10/1 -> Cross Product1/2
  Gain25/1 -> Add/8
  Demux1/2 -> Square1/1
  Gain18/1 -> Add/1
  Square2/1 -> Gain2/1
  Constant2/1 -> Cross Product2/1
  Constant3/1 -> Cross Product3/1
  Gain15/1 -> Add11/6
  Add1/1 -> T_F_b/1
  Demux1/7 -> Square6/1
  Gain2/1 -> Gain12/1
  Cross Product4/1 -> Gain21/1
  Demux2/6 -> Add1/6, MATLAB Function10/3(T_mot_in)
  Constant5/1 -> Cross Product5/1
  Demux1/1 -> Square/1
  Add7/1 -> Cross Product4/2
  Constant6/1 -> Cross Product6/1
  Constant1/1 -> Cross Product1/1
  Constant8/1 -> Cross Product8/1
  Demux2/1 -> Add1/1, MATLAB Function9/3(T_mot_in)
  Demux1/6 -> Square5/1
  Gain11/1 -> Add11/2
  Square/1 -> Gain/1
  Constant14/1 -> MATLAB Function7/1(phi)
  Constant19/1 -> MATLAB Function10/2(theta)
  Square7/1 -> Gain8/1
  Constant11/1 -> MATLAB Function5/2(theta)
  Demux1/5 -> Square4/1
  Demux2/7 -> Add1/7, MATLAB Function11/3(T_mot_in)
  Constant15/1 -> MATLAB Function7/2(theta)
  Gain12/1 -> Add11/3
  Mux/1 -> Add12/1
  Constant20/1 -> MATLAB Function11/1(phi)
  Square4/1 -> Gain5/1
  Add11/1 -> Mux/3
  Add6/1 -> Cross Product5/2
  MATLAB Function11/1(T_b_out) -> Add4/1
  MATLAB Function9/1(T_b_out) -> Add10/1
  Constant18/1 -> MATLAB Function10/1(phi)
  Add5/1 -> Cross Product6/2
  Gain/1 -> Gain9/1
  Add/1 -> Add12/2
  Gain6/1 -> Gain15/1
  Gain19/1 -> Add/2
  Gain22/1 -> Add/5
  Demux2/3 -> Add1/3, MATLAB Function6/3(T_mot_in)
  Constant13/1 -> MATLAB Function6/2(theta)
  Constant17/1 -> MATLAB Function8/2(theta)
  Gain8/1 -> Gain17/1
  MATLAB Function10/1(T_b_out) -> Add5/1
  Add3/1 -> Cross Product8/2
  Cross Product3/1 -> Gain20/1
  Gain14/1 -> Add11/5
  Square3/1 -> Gain4/1
  Constant21/1 -> MATLAB Function11/2(theta)
  Cross Product6/1 -> Gain23/1
  Constant26/1 -> Mux/1
  Gain21/1 -> Add/4
  Gain10/1 -> Demux1/1
  Cross Product2/1 -> Gain19/1
  Constant7/1 -> Cross Product7/1
  Demux1/3 -> Square2/1
  F_b_T/1 -> Demux2/1
  Gain1/1 -> Gain11/1
  Constant23/1 -> MATLAB Function12/2(theta)
  Gain7/1 -> Gain16/1
  MATLAB Function12/1(T_b_out) -> Add3/1
  Gain17/1 -> Add11/8
  Gain16/1 -> Add11/7
  Constant10/1 -> MATLAB Function5/1(phi)
  Gain9/1 -> Add11/1
  Add8/1 -> Cross Product3/2
  w_prop/1 -> Gain10/1
  Add9/1 -> Cross Product2/2
  Demux2/8 -> Add1/8, MATLAB Function12/3(T_mot_in)
  Add12/1 -> M_b_tot/1
  Square6/1 -> Gain7/1
  Constant9/1 -> MATLAB Function9/1(phi)
  Constant16/1 -> MATLAB Function8/1(phi)
  Demux1/8 -> Square7/1
  Gain4/1 -> Gain13/1
  Gain24/1 -> Add/7
  Cross Product1/1 -> Gain18/1
  Constant22/1 -> MATLAB Function12/1(phi)
  Cross Product8/1 -> Gain25/1
  Constant4/1 -> Cross Product4/1
  Constant12/1 -> MATLAB Function6/1(phi)
  Square1/1 -> Gain1/1
  Constant27/1 -> Mux/2
  MATLAB Function8/1(T_b_out) -> Add6/1
  MATLAB Function7/1(T_b_out) -> Add7/1
  MATLAB Function6/1(T_b_out) -> Add8/1
  Demux1/4 -> Square3/1
  Gain13/1 -> Add11/4
  Cross Product7/1 -> Gain24/1
  Cross Product5/1 -> Gain22/1
  Constant24/1 -> MATLAB Function9/2(theta)
  Square5/1 -> Gain6/1
  Gain5/1 -> Gain14/1
  Add4/1 -> Cross Product7/2
  Gain23/1 -> Add/6
  MATLAB Function5/1(T_b_out) -> Add9/1
  Demux2/2 -> Add1/2, MATLAB Function5/3(T_mot_in)
  Gain20/1 -> Add/3

== system Octacopter_Model_24b/Subsystem/Estimation/Subsystem3 ==
  In1 : Inport
  In2 : Inport  Port=2
  In3 : Inport  Port=3
  Bus Creator : BusCreator  Inputs=3
  Subsystem : Subsystem
  Subsystem1 : Subsystem
  Subsystem2 : Subsystem
  est_angular_rate : Outport
  wires:
  Bus Creator/1 -> est_angular_rate/1
  Subsystem/1(Out1) -> Bus Creator/1  "est_p"
  In3/1 -> Subsystem2/1(In1)
  In2/1 -> Subsystem1/1(In1)
  Subsystem2/1(Out1) -> Bus Creator/3  "est_r"
  Subsystem1/1(Out1) -> Bus Creator/2  "est_q"
  In1/1 -> Subsystem/1(In1)

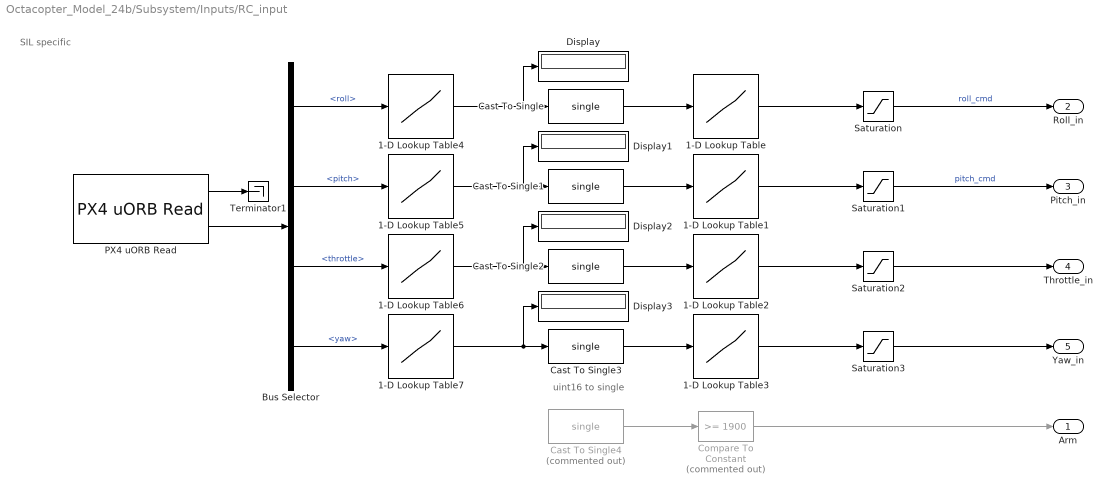
== system Octacopter_Model_24b/Subsystem/Inputs/RC_input ==
  note: uint16 to single
  note: SIL specific
  1-D Lookup Table : Lookup_n-D  NumberOfTableDimensions=1  BreakpointsForDimension1=([1000 1500 2000])  Table=single([-1 0 1])  InternalRulePriority=Speed  RndMeth=Simplest
  1-D Lookup Table1 : Lookup_n-D  NumberOfTableDimensions=1  BreakpointsForDimension1=([1000 1500 2000])  Table=single([-1 0 1])  InternalRulePriority=Speed  RndMeth=Simplest
  1-D Lookup Table2 : Lookup_n-D  NumberOfTableDimensions=1  BreakpointsForDimension1=([1000 1500 2000])  Table=single([0 0.5 1])  InternalRulePriority=Speed  RndMeth=Simplest
  1-D Lookup Table3 : Lookup_n-D  NumberOfTableDimensions=1  BreakpointsForDimension1=([1000 1500 2000])  Table=single([-1 0 1])  InternalRulePriority=Speed  RndMeth=Simplest
  1-D Lookup Table4 : Lookup_n-D  NumberOfTableDimensions=1  BreakpointsForDimension1=[-1, 0,1]  Table=single([1000, 1500, 2000])  InternalRulePriority=Speed  RndMeth=Simplest
  1-D Lookup Table5 : Lookup_n-D  NumberOfTableDimensions=1  BreakpointsForDimension1=[-1, 0,1]  Table=single([1000, 1500, 2000])  InternalRulePriority=Speed  RndMeth=Simplest
  1-D Lookup Table6 : Lookup_n-D  NumberOfTableDimensions=1  BreakpointsForDimension1=[0,1]  Table="single([1000,  2000])"  InternalRulePriority=Speed  RndMeth=Simplest
  1-D Lookup Table7 : Lookup_n-D  NumberOfTableDimensions=1  BreakpointsForDimension1=[-1, 0,1]  Table=single([1000, 1500, 2000])  InternalRulePriority=Speed  RndMeth=Simplest
  Bus Selector : BusSelector  OutputSignals=roll,pitch,throttle,yaw
  Cast To Single{,1..3} (4 alike) : DataTypeConversion  OutDataTypeStr=single  SaturateOnIntegerOverflow=off  RndMeth=Floor
  Cast To Single4 : DataTypeConversion  Commented=on  OutDataTypeStr=single  SaturateOnIntegerOverflow=off  RndMeth=Floor
  Compare To Constant : simulink/Logic and Bit Operations/Compare To Constant  Commented=on  relop=>=  const=1900  OutDataTypeStr=boolean
  Display{,1..3} (4 alike) : Display
  PX4 uORB Read : px4uORBlib/PX4 uORB Read  uORBTopic=ManualControlSetpoint  selectInstance=manual_control_setpoint  SampleTime=0.001  BlockingMode=off  BlockTimeout=1e-3
  Saturation : Saturate  UpperLimit=1  LowerLimit=-1
  Saturation1 : Saturate  UpperLimit=1  LowerLimit=-1
  Saturation2 : Saturate  UpperLimit=1  LowerLimit=0
  Saturation3 : Saturate  UpperLimit=1  LowerLimit=-1
  Terminator1 : Terminator
  Arm : Outport
  Roll_in : Outport  Port=2
  Pitch_in : Outport  Port=3
  Throttle_in : Outport  Port=4
  Yaw_in : Outport  Port=5
  wires:
  Compare To Constant/1 -> Arm/1
  Bus Selector/3 -> 1-D Lookup Table6/1  "<throttle>"
  Saturation3/1 -> Yaw_in/1
  Cast To Single/1 -> 1-D Lookup Table/1
  Saturation2/1 -> Throttle_in/1
  Bus Selector/2 -> 1-D Lookup Table5/1  "<pitch>"
  Cast To Single1/1 -> 1-D Lookup Table1/1
  Cast To Single3/1 -> 1-D Lookup Table3/1
  Cast To Single4/1 -> Compare To Constant/1
  Cast To Single2/1 -> 1-D Lookup Table2/1
  Saturation1/1 -> Pitch_in/1  "pitch_cmd"
  Saturation/1 -> Roll_in/1  "roll_cmd"
  1-D Lookup Table/1 -> Saturation/1
  1-D Lookup Table1/1 -> Saturation1/1
  1-D Lookup Table2/1 -> Saturation2/1
  1-D Lookup Table3/1 -> Saturation3/1
  Bus Selector/4 -> 1-D Lookup Table7/1  "<yaw>"
  Bus Selector/1 -> 1-D Lookup Table4/1  "<roll>"
  PX4 uORB Read/2 -> Bus Selector/1
  PX4 uORB Read/1 -> Terminator1/1
  1-D Lookup Table4/1 -> Display/1, Cast To Single/1
  1-D Lookup Table5/1 -> Display1/1, Cast To Single1/1
  1-D Lookup Table7/1 -> Display3/1, Cast To Single3/1
  1-D Lookup Table6/1 -> Display2/1, Cast To Single2/1

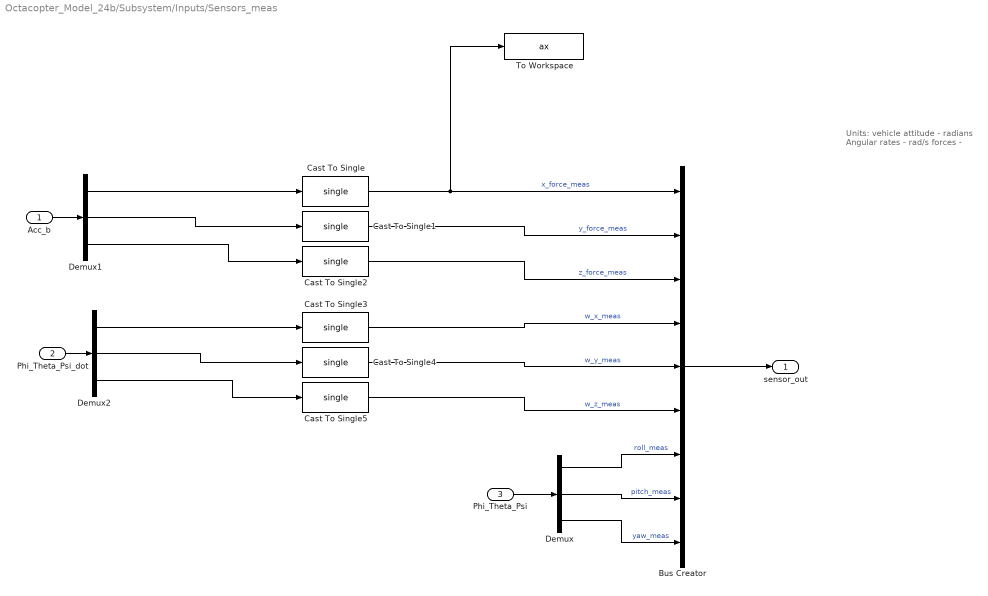
== system Octacopter_Model_24b/Subsystem/Inputs/Sensors_meas ==
  note: Units:
      | vehicle attitude - radians
      | Angular rates - rad/s
      | forces -
  Acc_b : Inport
  Phi_Theta_Psi_dot : Inport  Port=2
  Phi_Theta_Psi : Inport  Port=3
  Bus Creator : BusCreator  Inputs=9
  Cast To Single{,1..5} (6 alike) : DataTypeConversion  OutDataTypeStr=single  SaturateOnIntegerOverflow=off  RndMeth=Floor
  Demux : Demux  Outputs=3
  Demux1 : Demux  Outputs=3
  Demux2 : Demux  Outputs=3
  To Workspace : ToWorkspace  VariableName=ax  SaveFormat=Structure With Time  SampleTime=-1
  sensor_out : Outport
  wires:
  Demux2/1 -> Cast To Single3/1
  Cast To Single4/1 -> Bus Creator/5  "w_y_meas"
  Demux1/1 -> Cast To Single/1
  Demux/1 -> Bus Creator/7  "roll_meas"
  Demux/2 -> Bus Creator/8  "pitch_meas"
  Demux/3 -> Bus Creator/9  "yaw_meas"
  Demux2/3 -> Cast To Single5/1
  Cast To Single5/1 -> Bus Creator/6  "w_z_meas"
  Bus Creator/1 -> sensor_out/1
  Demux1/2 -> Cast To Single1/1
  Cast To Single/1 -> To Workspace/1, Bus Creator/1  "x_force_meas"
  Demux1/3 -> Cast To Single2/1
  Phi_Theta_Psi/1 -> Demux/1
  Cast To Single3/1 -> Bus Creator/4  "w_x_meas"
  Cast To Single1/1 -> Bus Creator/2  "y_force_meas"
  Cast To Single2/1 -> Bus Creator/3  "z_force_meas"
  Acc_b/1 -> Demux1/1
  Phi_Theta_Psi_dot/1 -> Demux2/1
  Demux2/2 -> Cast To Single4/1

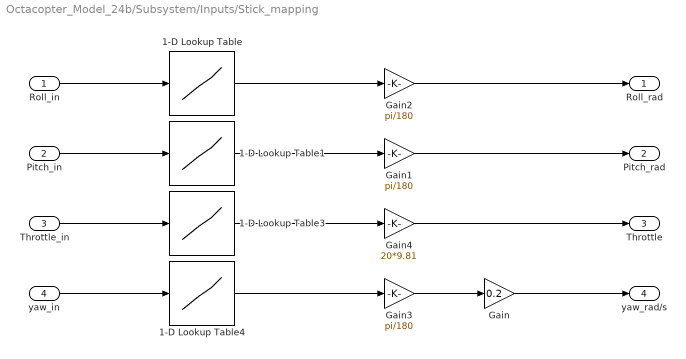
== system Octacopter_Model_24b/Subsystem/Inputs/Stick_mapping ==
  Roll_in : Inport
  Pitch_in : Inport  Port=2
  Throttle_in : Inport  Port=3
  yaw_in : Inport  Port=4
  1-D Lookup Table : Lookup_n-D  NumberOfTableDimensions=1  BreakpointsForDimension1=single([-1,1])  Table=single([-30,30])  InternalRulePriority=Speed  RndMeth=Simplest
  1-D Lookup Table1 : Lookup_n-D  NumberOfTableDimensions=1  BreakpointsForDimension1=single([-1,1])  Table=single([30,-30])  InternalRulePriority=Speed  RndMeth=Simplest
  1-D Lookup Table3 : Lookup_n-D  NumberOfTableDimensions=1  BreakpointsForDimension1=single([0 0.100000001 0.25 0.5 0.75 1])  Table=single([0 -0.200000003 -0.5 -1 -1.5 -2])  InternalRulePriority=Speed  RndMeth=Simplest
  1-D Lookup Table4 : Lookup_n-D  NumberOfTableDimensions=1  BreakpointsForDimension1=single([-1,1])  Table=single([-90,90])  InternalRulePriority=Speed  RndMeth=Simplest
  Gain : Gain  Gain=0.2
  Gain1 : Gain  Gain=pi/180
  Gain2 : Gain  Gain=pi/180
  Gain3 : Gain  Gain=pi/180
  Gain4 : Gain  Gain=20*9.81
  Roll_rad : Outport
  Pitch_rad : Outport  Port=2
  Throttle : Outport  Port=3
  yaw_rad/s : Outport  Port=4
  wires:
  Gain1/1 -> Pitch_rad/1
  Roll_in/1 -> 1-D Lookup Table/1
  Pitch_in/1 -> 1-D Lookup Table1/1
  yaw_in/1 -> 1-D Lookup Table4/1
  Throttle_in/1 -> 1-D Lookup Table3/1
  1-D Lookup Table1/1 -> Gain1/1
  1-D Lookup Table/1 -> Gain2/1
  1-D Lookup Table3/1 -> Gain4/1
  1-D Lookup Table4/1 -> Gain3/1
  Gain2/1 -> Roll_rad/1
  Gain3/1 -> Gain/1
  Gain4/1 -> Throttle/1
  Gain/1 -> yaw_rad/s/1

== system Octacopter_Model_24b/Subsystem/PI_controller /Subsystem ==
  phi_cmd : Inport
  theta_cmd : Inport  Port=2
  psi_cmd : Inport  Port=3
  est_att : Inport  Port=4
  Bus Selector : BusSelector  OutputSignals=roll,pitch
  Inverse_strapdown : Subsystem
  Signal Copy : SignalConversion  OverrideOpt=off
  Sum : Sum  Inputs=|+-
  Sum1 : Sum  Inputs=|+-
  phi_err_gain : Gain  Gain=0.7133389565007833
  theta_err_gain : Gain  Gain=0.7075551271237498
  p_cmd : Outport
  q_cmd : Outport  Port=2
  r_dot_cmd : Outport  Port=3
  wires:
  Bus Selector/2 -> Inverse_strapdown/4(est_theta), Sum1/2  "<pitch>"
  Bus Selector/1 -> Sum/2, Inverse_strapdown/3(est_phi)  "<roll>"
  Sum1/1 -> theta_err_gain/1  "theta_error"
  theta_cmd/1 -> Sum1/1
  phi_cmd/1 -> Sum/1
  Sum/1 -> phi_err_gain/1  "phi_error"
  psi_cmd/1 -> Signal Copy/1  "psi_cmd"
  Signal Copy/1 -> Inverse_strapdown/5(psi_dot_cmd)  "psi_dot_cmd"
  theta_err_gain/1 -> Inverse_strapdown/2(theta_dot_cmd)
  phi_err_gain/1 -> Inverse_strapdown/1(phi_dot_cmd)
  est_att/1 -> Bus Selector/1
  Inverse_strapdown/1(p_cmd) -> p_cmd/1
  Inverse_strapdown/2(q_cmd) -> q_cmd/1
  Inverse_strapdown/3(r_dot_cmd) -> r_dot_cmd/1

== system Octacopter_Model_24b/Subsystem/PI_controller /rotational ==
  p_cmd : Inport
  q_cmd : Inport  Port=2
  r_dot_cmd : Inport  Port=3
  est_angular_rate : Inport  Port=4
  Bus Selector : BusSelector  OutputSignals=est_p,est_q
  Pitch_PID : Subsystem
  Roll_PID : Subsystem
  Sum : Sum  Inputs=|+-
  Sum1 : Sum  Inputs=|+-
  P_dot : Outport
  q_dot : Outport  Port=2
  r_dot : Outport  Port=3
  wires:
  Sum/1 -> Roll_PID/1(Roll_error)  "p_error"
  Sum1/1 -> Pitch_PID/1(Pitch_error)  "q_error"
  Roll_PID/1(phi_dot) -> P_dot/1
  Bus Selector/2 -> Sum1/2  "<est_q>"
  p_cmd/1 -> Sum/1
  Pitch_PID/1(Theta_dot) -> q_dot/1
  r_dot_cmd/1 -> r_dot/1
  q_cmd/1 -> Sum1/1
  Bus Selector/1 -> Sum/2  "<est_p>"
  est_angular_rate/1 -> Bus Selector/1

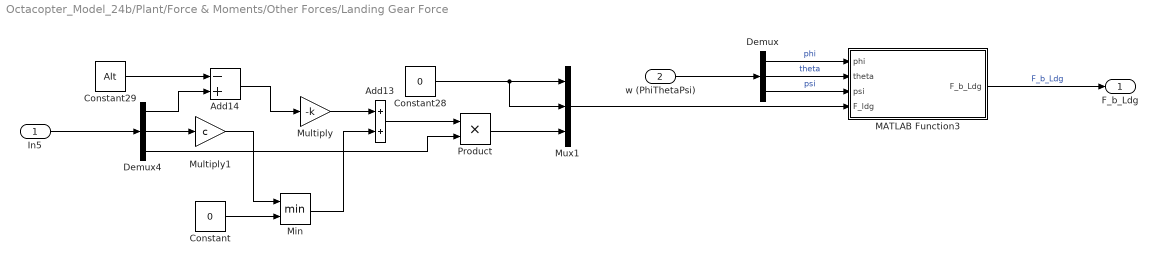
== system Octacopter_Model_24b/Plant/Force & Moments/Other Forces/Landing Gear Force ==
  In5 : Inport
  w (PhiThetaPsi) : Inport  Port=2
  Add13 : Sum
  Add14 : Sum  Inputs=-+
  Constant : Constant  Value=0
  Constant28 : Constant  Value=0
  Constant29 : Constant  Value=Alt
  Demux : Demux  Outputs=3
  Demux4 : Demux  Outputs=3
  MATLAB Function3 : MATLAB Function  TreatAsAtomicUnit=on
  Min : MinMax  Inputs=2
  Multiply : Gain  Gain=-k
  Multiply1 : Gain  Gain=c
  Mux1 : Mux  Inputs=3
  Product : Product
  F_b_Ldg : Outport
  wires:
  Product/1 -> Mux1/3
  Add13/1 -> Product/1
  Demux4/1 -> Add14/2
  Multiply1/1 -> Min/1
  In5/1 -> Demux4/1
  Multiply/1 -> Add13/1
  Constant28/1 -> Mux1/1, Mux1/2
  Demux4/2 -> Multiply1/1
  Demux4/3 -> Product/2
  Constant29/1 -> Add14/1
  Add14/1 -> Multiply/1
  Mux1/1 -> MATLAB Function3/4(F_ldg)
  Demux/2 -> MATLAB Function3/2(theta)  "theta"
  Demux/1 -> MATLAB Function3/1(phi)  "phi"
  w (PhiThetaPsi)/1 -> Demux/1
  Demux/3 -> MATLAB Function3/3(psi)  "psi"
  MATLAB Function3/1(F_b_Ldg) -> F_b_Ldg/1  "F_b_Ldg"
  Constant/1 -> Min/2
  Min/1 -> Add13/2

== system Octacopter_Model_24b/Subsystem/Estimation/Subsystem3/Subsystem ==
  In1 : Inport
  DI : Subsystem
  Gain : Gain  Gain=0.6270996640537514
  Saturation1 : Saturate  UpperLimit=5.24  LowerLimit=-5.24
  Sum : Sum  Inputs=|+-
  Out1 : Outport
  wires:
  Sum/1 -> Gain/1
  Gain/1 -> DI/1(In1)
  DI/1(Out1) -> Saturation1/1, Sum/2
  In1/1 -> DI/2(In2), Sum/1
  Saturation1/1 -> Out1/1

== system Octacopter_Model_24b/Subsystem/Estimation/Subsystem3/Subsystem1 ==
  In1 : Inport
  DI : Subsystem
  Gain : Gain  Gain=0.6382978723404255
  Saturation1 : Saturate  UpperLimit=5.24  LowerLimit=-5.24
  Sum : Sum  Inputs=|+-
  Out1 : Outport
  wires:
  Sum/1 -> Gain/1
  DI/1(Out1) -> Saturation1/1, Sum/2
  Gain/1 -> DI/1(In1)
  In1/1 -> DI/2(In2), Sum/1
  Saturation1/1 -> Out1/1

== system Octacopter_Model_24b/Subsystem/Estimation/Subsystem3/Subsystem2 ==
  In1 : Inport
  DI : Subsystem
  Gain : Gain  Gain=0.6606942889137737
  Saturation1 : Saturate  UpperLimit=5.24  LowerLimit=-5.24
  Sum : Sum  Inputs=|+-
  Out1 : Outport
  wires:
  Sum/1 -> Gain/1
  DI/1(Out1) -> Saturation1/1, Sum/2
  Gain/1 -> DI/1(In1)
  In1/1 -> DI/2(In2), Sum/1
  Saturation1/1 -> Out1/1

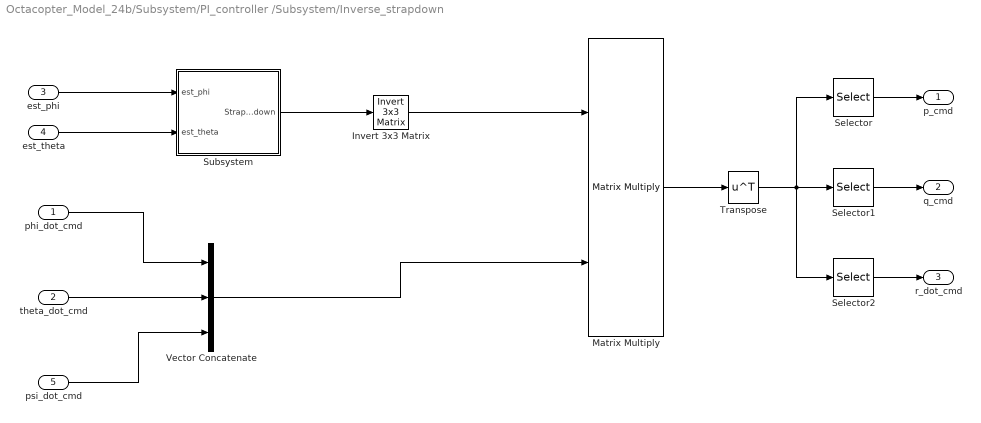
== system Octacopter_Model_24b/Subsystem/PI_controller /Subsystem/Inverse_strapdown ==
  phi_dot_cmd : Inport
  theta_dot_cmd : Inport  Port=2
  est_phi : Inport  Port=3
  est_theta : Inport  Port=4
  psi_dot_cmd : Inport  Port=5
  Invert 3x3 Matrix : aerolibutil/Invert  3x3 Matrix
  Matrix Multiply : Product  Multiplication=Matrix(*)
  Selector : Selector  InputPortWidth=3  IndexOptions=Index vector (dialog)  Indices=1  OutputSizes=1
  Selector1 : Selector  InputPortWidth=3  IndexOptions=Index vector (dialog)  Indices=2  OutputSizes=1
  Selector2 : Selector  InputPortWidth=3  IndexOptions=Index vector (dialog)  Indices=3  OutputSizes=1
  Subsystem : Subsystem
  Transpose : Math  Operator=transpose
  Vector Concatenate : Concatenate  NumInputs=3  Mode=Multidimensional array
  p_cmd : Outport
  q_cmd : Outport  Port=2
  r_dot_cmd : Outport  Port=3
  wires:
  Vector Concatenate/1 -> Matrix Multiply/2
  Subsystem/1(Strap_down) -> Invert 3x3 Matrix/1
  Invert 3x3 Matrix/1 -> Matrix Multiply/1
  est_phi/1 -> Subsystem/1(est_phi)
  est_theta/1 -> Subsystem/2(est_theta)
  Matrix Multiply/1 -> Transpose/1
  Transpose/1 -> Selector2/1, Selector1/1, Selector/1
  Selector/1 -> p_cmd/1
  Selector1/1 -> q_cmd/1
  Selector2/1 -> r_dot_cmd/1
  phi_dot_cmd/1 -> Vector Concatenate/1
  theta_dot_cmd/1 -> Vector Concatenate/2
  psi_dot_cmd/1 -> Vector Concatenate/3

== system Octacopter_Model_24b/Subsystem/PI_controller /rotational/Pitch_PID ==
  Pitch_error : Inport
  Discrete-Time Integrator : DiscreteIntegrator  SampleTime=-1  ICPrevOutput=DiscIntNeverNeededParam  ICPrevScaledInput=DiscIntNeverNeededParam
  Display : Display
  I_pitch : Gain  Gain=single(0.01985781)
  P_pitch : Gain  Gain=0.1306122448979592
  Sum : Sum  Inputs=|++
  Theta_dot : Outport
  wires:
  Sum/1 -> Display/1, Theta_dot/1
  Discrete-Time Integrator/1 -> I_pitch/1
  P_pitch/1 -> Sum/1
  Pitch_error/1 -> Discrete-Time Integrator/1, P_pitch/1
  I_pitch/1 -> Sum/2

== system Octacopter_Model_24b/Subsystem/PI_controller /rotational/Roll_PID ==
  Roll_error : Inport
  Discrete-Time Integrator : DiscreteIntegrator  gainval=1  SampleTime=-1  ICPrevOutput=DiscIntNeverNeededParam  ICPrevScaledInput=DiscIntNeverNeededParam
  Display : Display
  Display1 : Display
  Display2 : Display
  I_roll : Gain  Gain=0.01999448681429753
  P_roll : Gain  Gain=0.1445180189801959
  Sum : Sum  Inputs=|++
  phi_dot : Outport
  wires:
  Sum/1 -> phi_dot/1
  P_roll/1 -> Display/1, Sum/1
  I_roll/1 -> Discrete-Time Integrator/1  "int_err_unsat"
  Discrete-Time Integrator/1 -> Sum/2, Display2/1
  Roll_error/1 -> Display1/1, I_roll/1, P_roll/1

== system Octacopter_Model_24b/Subsystem/Estimation/Subsystem3/Subsystem/DI ==
  In1 : Inport
  In2 : Inport  Port=2
  Constant2 : Constant  Value=0.004
  Divide : Product  Inputs=*/
  Gain : Gain  Gain=0.004*2
  Step : Step  Time=0.02  Before=1  After=0  SampleTime=0.004
  Sum : Sum  Inputs=|++
  Sum1 : Sum  Inputs=|++
  Switch : Switch  Criteria=u2 > Threshold  SaturateOnIntegerOverflow=off  InputSameDT=off
  Unit Delay : UnitDelay  SampleTime=-1  HasFrameUpgradeWarning=on
  Out1 : Outport
  wires:
  Step/1 -> Switch/2
  Sum1/1 -> Unit Delay/1
  Divide/1 -> Switch/1
  Switch/1 -> Sum1/2, Sum/2, Sum/1
  Sum/1 -> Gain/1
  Constant2/1 -> Divide/2
  Gain/1 -> Out1/1
  In1/1 -> Sum1/1
  In2/1 -> Divide/1
  Unit Delay/1 -> Switch/3

== system Octacopter_Model_24b/Subsystem/Estimation/Subsystem3/Subsystem1/DI ==
  In1 : Inport
  In2 : Inport  Port=2
  Constant2 : Constant  Value=0.004
  Divide : Product  Inputs=*/
  Gain : Gain  Gain=0.004*2
  Step : Step  Time=0.02  Before=1  After=0  SampleTime=0.004
  Sum : Sum  Inputs=|++
  Sum1 : Sum  Inputs=|++
  Switch : Switch  Criteria=u2 > Threshold  SaturateOnIntegerOverflow=off  InputSameDT=off
  Unit Delay : UnitDelay  SampleTime=-1  HasFrameUpgradeWarning=on
  Out1 : Outport
  wires:
  Step/1 -> Switch/2
  Sum1/1 -> Unit Delay/1
  Unit Delay/1 -> Switch/3
  Divide/1 -> Switch/1
  Switch/1 -> Sum1/2, Sum/2, Sum/1
  Sum/1 -> Gain/1
  Constant2/1 -> Divide/2
  Gain/1 -> Out1/1
  In1/1 -> Sum1/1
  In2/1 -> Divide/1

== system Octacopter_Model_24b/Subsystem/Estimation/Subsystem3/Subsystem2/DI ==
  In1 : Inport
  In2 : Inport  Port=2
  Constant2 : Constant  Value=0.004
  Divide : Product  Inputs=*/
  Gain : Gain  Gain=0.004*2
  Step : Step  Time=0.02  Before=1  After=0  SampleTime=0.004
  Sum : Sum  Inputs=|++
  Sum1 : Sum  Inputs=|++
  Switch : Switch  Criteria=u2 > Threshold  SaturateOnIntegerOverflow=off  InputSameDT=off
  Unit Delay : UnitDelay  SampleTime=-1  HasFrameUpgradeWarning=on
  Out1 : Outport
  wires:
  Step/1 -> Switch/2
  Sum1/1 -> Unit Delay/1
  Unit Delay/1 -> Switch/3
  Divide/1 -> Switch/1
  Switch/1 -> Sum1/2, Sum/2, Sum/1
  Sum/1 -> Gain/1
  Constant2/1 -> Divide/2
  Gain/1 -> Out1/1
  In1/1 -> Sum1/1
  In2/1 -> Divide/1

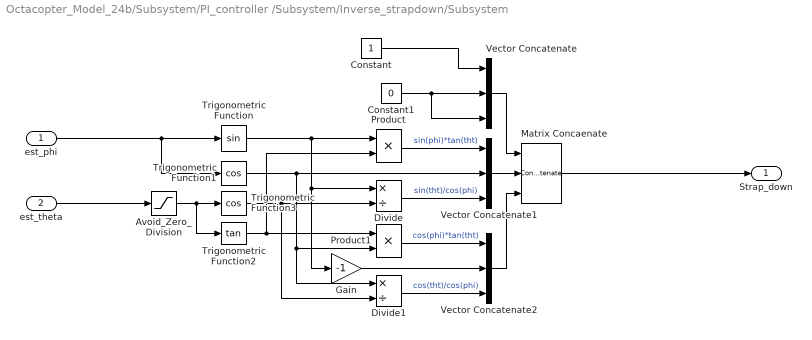
== system Octacopter_Model_24b/Subsystem/PI_controller /Subsystem/Inverse_strapdown/Subsystem ==
  est_phi : Inport
  est_theta : Inport  Port=2
  Avoid_Zero_Division : Saturate  UpperLimit=pi/2*0.9  LowerLimit=-pi/2*0.9
  Constant : Constant  OutDataTypeStr=single
  Constant1 : Constant  Value=0  OutDataTypeStr=single
  Divide : Product  Inputs=*/
  Divide1 : Product  Inputs=*/
  Gain : Gain  Gain=-1
  Matrix Concaenate : Concatenate  NumInputs=3  Mode=Multidimensional array  ConcatenateDimension=2
  Product : Product  RndMeth=Zero
  Product1 : Product  RndMeth=Zero
  Trigonometric Function : Trigonometry
  Trigonometric Function1 : Trigonometry  Operator=cos
  Trigonometric Function2 : Trigonometry  Operator=tan
  Trigonometric Function3 : Trigonometry  Operator=cos
  Vector Concatenate : Concatenate  NumInputs=3  Mode=Multidimensional array
  Vector Concatenate1 : Concatenate  NumInputs=3  Mode=Multidimensional array
  Vector Concatenate2 : Concatenate  NumInputs=3  Mode=Multidimensional array
  Strap_down : Outport
  wires:
  Vector Concatenate1/1 -> Matrix Concaenate/2
  Product1/1 -> Vector Concatenate2/1  "cos(phi)*tan(tht)"
  Trigonometric Function1/1 -> Vector Concatenate1/2, Divide1/1, Product1/2
  est_phi/1 -> Trigonometric Function1/1, Trigonometric Function/1
  Constant1/1 -> Vector Concatenate/2, Vector Concatenate/3
  Trigonometric Function3/1 -> Divide/2, Divide1/2
  Avoid_Zero_Division/1 -> Trigonometric Function3/1, Trigonometric Function2/1
  Gain/1 -> Vector Concatenate2/2
  Divide/1 -> Vector Concatenate1/3  "sin(tht)/cos(phi)"
  Vector Concatenate2/1 -> Matrix Concaenate/3
  Divide1/1 -> Vector Concatenate2/3  "cos(tht)/cos(phi)"
  est_theta/1 -> Avoid_Zero_Division/1
  Product/1 -> Vector Concatenate1/1  "sin(phi)*tan(tht)"
  Vector Concatenate/1 -> Matrix Concaenate/1
  Constant/1 -> Vector Concatenate/1
  Matrix Concaenate/1 -> Strap_down/1
  Trigonometric Function2/1 -> Product/2, Product1/1
  Trigonometric Function/1 -> Product/1, Divide/1, Gain/1
